simulink model "PTB_GliderModel"  (R2018a)
settings: Solver=ode23tb  StartTime=0.0  StopTime=TimeUS06  RelTol=1e-3
model workspace (MAT data in the model file):
  Af = 4
  Cd = 0.3
  D = 0.322411602927
  DrCycles.C505 = [0 1 2 3 4 5 6 7 8 9 10 11 ... (1012 elements, 506x2)]
  DrCycles.FTP = [0 1 2 3 4 5 6 7 8 9 10 11 ... (4956 elements, 2478x2)]
  DrCycles.UDDS = [0 1 2 3 4 5 6 7 8 9 10 11 ... (2746 elements, 1373x2)]
  DrCycles.HWFET = [0 1 2 3 4 5 6 7 8 9 10 11 ... (1532 elements, 766x2)]
  DrCycles.US06 = [0 1 2 3 4 5 6 7 8 9 10 11 ... (1194 elements, 597x2)]
  DrCycles.US06City = [0 1 2 3 4 5 6 7 8 9 10 11 ... (466 elements, 233x2)]
  DrCycles.US06Hwy = [0 1 2 3 4 5 6 7 8 9 10 11 ... (742 elements, 371x2)]
  I = 0.017709310577
  Kbr = 5000
  P = 1716.45095687
  TimeHWFET = 765
  TimeUDDS = 1372
  TimeUS06 = 596
  vehicleMass = 1500
  wheelRadius = 0.35
libraries: Wheels_Driver_VehDyn_Lib x2, simulink x1
settings Model: Creator=emarquez  LastModifiedBy=emarquez
settings DebuggingCC: AlgebraicLoopMsg=none
settings CodeAppCC: StateflowObjectComments=on
settings SimscapeCC: SimscapeNormalizeSystem=off

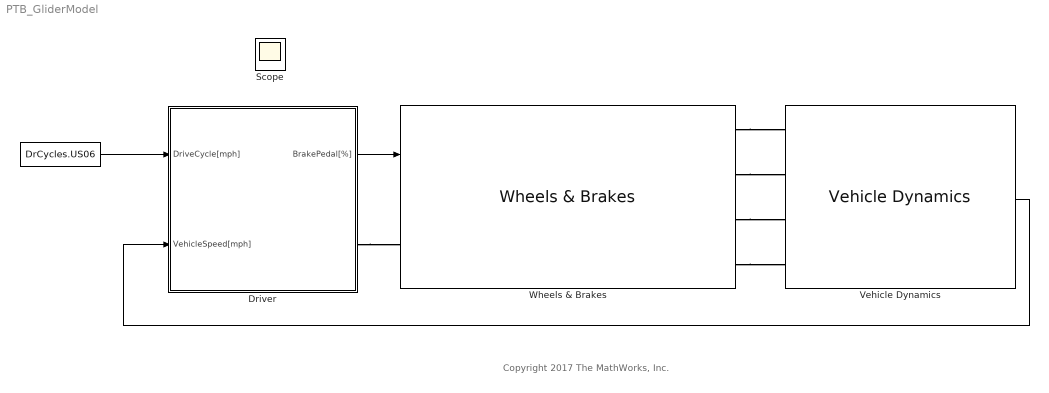
== system PTB_GliderModel ==
  note: Copyright 2017 The MathWorks, Inc.
  " " : FromWorkspace  Tag=DriveCycle  VariableName=DrCycles.US06  SampleTime=0
  Driver : Subsystem
  Vehicle Dynamics : Wheels_Driver_VehDyn_Lib/Vehicle Dynamics
  Wheels & Brakes : Wheels_Driver_VehDyn_Lib/Wheels & Brakes
  Scope : Scope
  wires:
  " "/1 -> Driver/1(" DriveCycle[mph]")
  Vehicle Dynamics/1 -> Driver/2(VehicleSpeed[mph])
  Driver/1(BrakePedal[%]) -> Wheels & Brakes/1
  connections:
  Wheels & Brakes/RConn3 -- Vehicle Dynamics/LConn3
  Wheels & Brakes/RConn4 -- Vehicle Dynamics/LConn4
  Wheels & Brakes/RConn2 -- Vehicle Dynamics/LConn2
  Wheels & Brakes/RConn1 -- Vehicle Dynamics/LConn1
  Driver/RConn1 -- Wheels & Brakes/LConn1

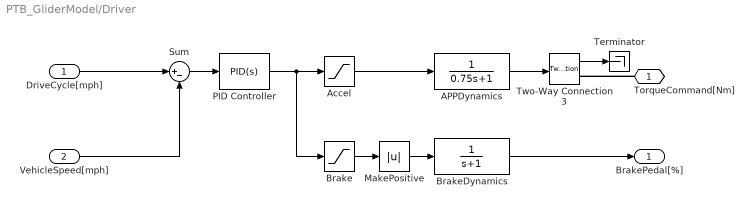
== system PTB_GliderModel/Driver ==
  " DriveCycle[mph]" : Inport
  VehicleSpeed[mph] : Inport  Port=2
  APPDynamics : TransferFcn  Denominator=[0.75 1]
  Accel : Saturate  UpperLimit=inf  LowerLimit=0
  Brake : Saturate  UpperLimit=0  LowerLimit=-100
  BrakeDynamics : TransferFcn  Denominator=[1 1]
  MakePositive : Abs
  PID Controller : simulink/Continuous/PID Controller  Controller=PID  TimeDomain=Continuous-time  SampleTime=-1  IntegratorMethod=Forward Euler  FilterMethod=Forward Euler  Form=Parallel  UseFilter=on  ControllerParametersSource=internal  P=P  I=I  D=D  N=100  InitialConditionSource=internal  InitialConditionForIntegrator=0  InitialConditionForFilter=0  ExternalReset=none  LimitOutput=on  UpperSaturationLimit=inf  LowerSaturationLimit=-100  LinearizeAsGain=on  AntiWindupMode=none  Kb=1  TrackingMode=off  Kt=1  PParamMin=[]  PParamMax=[]  IParamMin=[]  IParamMax=[]  DParamMin=[]  DParamMax=[]  NParamMin=[]  NParamMax=[]  KbParamMin=[]  KbParamMax=[]  KtParamMin=[]  KtParamMax=[]  POutMin=[]  POutMax=[]  IOutMin=[]  IOutMax=[]  DOutMin=[]  DOutMax=[]  NOutMin=[]  NOutMax=[]  KbOutMin=[]  KbOutMax=[]  KtOutMin=[]  KtOutMax=[]  IntegratorOutMin=[]  IntegratorOutMax=[]  FilterOutMin=[]  FilterOutMax=[]  SumOutMin=[]  SumOutMax=[]  SumI1OutMin=[]  SumI1OutMax=[]  SumI2OutMin=[]  SumI2OutMax=[]  SumI3OutMin=[]  SumI3OutMax=[]  SumDOutMin=[]  SumDOutMax=[]  SaturationOutMin=[]  SaturationOutMax=[]  IntegratorContinuousStateAttributes=''  IntegratorStateMustResolveToSignalObject=off  IntegratorRTWStateStorageClass=Auto  FilterContinuousStateAttributes=''  FilterStateMustResolveToSignalObject=off  FilterRTWStateStorageClass=Auto  DifferentiatorICPrevScaledInput=0  DifferentiatorOutMin=[]  DifferentiatorOutMax=[]  InitialConditionSetting=State (most efficient)  FilterDiffOutCoefMin=[]  FilterDiffOutCoefMax=[]  SumDenOutMin=[]  SumDenOutMax=[]  SumNumOutMin=[]  SumNumOutMax=[]  ReciprocalOutMin=[]  ReciprocalOutMax=[]  DivideOutMin=[]  DivideOutMax=[]  TunerSelectOption=Transfer Function Based (PID Tuner App)
  Sum : Sum  Inputs=|+-
  Terminator : Terminator
  Two-Way Connection3 : TwoWayConnection
  TorqueCommand[Nm] : PMIOPort  Side=Right
  BrakePedal[%] : Outport
  wires:
  MakePositive/1 -> BrakeDynamics/1
  BrakeDynamics/1 -> BrakePedal[%]/1
  " DriveCycle[mph]"/1 -> Sum/1
  VehicleSpeed[mph]/1 -> Sum/2
  PID Controller/1 -> Accel/1, Brake/1
  Sum/1 -> PID Controller/1
  Brake/1 -> MakePositive/1
  Accel/1 -> APPDynamics/1
  Two-Way Connection3/1 -> Terminator/1
  APPDynamics/1 -> Two-Way Connection3/1
  connections:
  TorqueCommand[Nm]/RConn1 -- Two-Way Connection3/RConn1
